simulink model "Open_Loop_shift"  (R2015a)
settings: Solver=ode3  StartTime=0.0  StopTime=300  FixedStep=0.01  MaxStep=0.01  RelTol=1e-3
values from neighbouring files (symbols this model uses):
  H0 = Periodic_Solution(1,4)    [Optimal_Entrainment_shiftworker.m]
  Ishift = 1000    [Optimal_Entrainment_shiftworker.m]
  n0 = Periodic_Solution(1,7)    [Optimal_Entrainment_shiftworker.m]
  Periodic_Solution = Periodic_Solution(1401:end,:)    [Optimal_Entrainment_shiftworker.m]
  shift = 12    [Optimal_Entrainment_shiftworker.m]
  tol = 0.01    [Optimal_Entrainment_shiftworker.m]
  x0 = Periodic_Solution(1,2)    [Optimal_Entrainment_shiftworker.m]
  xc0 = Periodic_Solution(1,3)    [Optimal_Entrainment_shiftworker.m]
settings Model: Creator=wangf7  LastModifiedBy=Jiawei Yin
settings OptimizationCC: ExpressionDepthLimit=2147483647
settings DebuggingCC: AlgebraicLoopMsg=none  ArtificialAlgebraicLoopMsg=none  UnderspecifiedInitializationDetection=Classic  MergeDetectMultiDrivingBlocksExec=none  SolverPrmCheckMsg=warning  StateNameClashWarn=warning

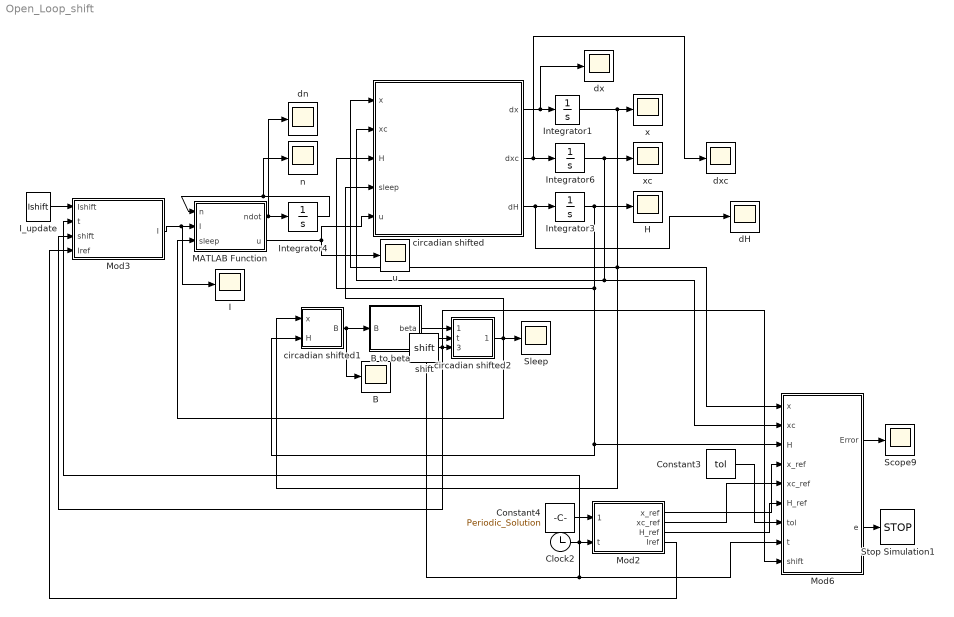
== system Open_Loop_shift ==
  B : Scope
      settings: TimeRange=auto  MaxDataPoints=5000  SaveName=B  YMin=-10  YMax=10  SampleTime=-1  DataFormat=Array
  "B to beta " : Subsystem
  Clock2 : Clock
  Constant3 : Constant  Value=tol
  Constant4 : Constant  Value=Periodic_Solution
  H : Scope
      settings: TimeRange=auto  MaxDataPoints=5000  SaveName=H  YMin=0.08394  YMax=0.57854  SampleTime=-1  DataFormat=Array
  I : Scope
      settings: TimeRange=auto  MaxDataPoints=5000  SaveName=I  YMin=-125.00000  YMax=1125.00000  SampleTime=-1  DataFormat=Array
  I_update : Constant  Value=Ishift
  Integrator1 : Integrator  InitialCondition=x0
  Integrator3 : Integrator  InitialCondition=H0
  Integrator4 : Integrator  InitialCondition=n0
  Integrator6 : Integrator  InitialCondition=xc0
  MATLAB Function : MATLAB Function  TreatAsAtomicUnit=on
      settings: PermitHierarchicalResolution=ParametersOnly
  Mod2 : MATLAB Function  TreatAsAtomicUnit=on
      settings: PermitHierarchicalResolution=ParametersOnly
  Mod3 : MATLAB Function  TreatAsAtomicUnit=on
      settings: PermitHierarchicalResolution=ParametersOnly
  Mod6 : MATLAB Function  TreatAsAtomicUnit=on
      settings: PermitHierarchicalResolution=ParametersOnly
  Scope9 : Scope
      settings: TimeRange=auto  MaxDataPoints=5000  SaveName=Error  YMin=0.00087  YMax=0.09507  SampleTime=-1  DataFormat=Array
  Sleep : Scope
      settings: TimeRange=auto  MaxDataPoints=5000  SaveName=Sleep  YMin=-0.125  YMax=1.125  SampleTime=-1  DataFormat=Array
  Stop Simulation1 : Stop
  circadian shifted : MATLAB Function  TreatAsAtomicUnit=on
      settings: PermitHierarchicalResolution=ParametersOnly
  circadian shifted1 : MATLAB Function  TreatAsAtomicUnit=on
      settings: PermitHierarchicalResolution=ParametersOnly
  circadian shifted2 : MATLAB Function  TreatAsAtomicUnit=on
      settings: PermitHierarchicalResolution=ParametersOnly
  dH : Scope
      settings: TimeRange=auto  MaxDataPoints=5000  SaveName=dH  YMin=0.03966  YMax=0.05966  SampleTime=-1  DataFormat=Array
  dn : Scope
      settings: TimeRange=auto  MaxDataPoints=5000  SaveName=dn  YMin=-10  YMax=10  SampleTime=-1  DataFormat=Array
  dx : Scope
      settings: TimeRange=auto  MaxDataPoints=5000  SaveName=dx  YMin=-10  YMax=10  SampleTime=-1  DataFormat=Array
  dxc : Scope
      settings: TimeRange=auto  MaxDataPoints=5000  SaveName=dxc  YMin=-10  YMax=10  SampleTime=-1  DataFormat=Array
  n : Scope
      settings: TimeRange=auto  MaxDataPoints=5000  SaveName=n  YMin=-10  YMax=10  SampleTime=-1  DataFormat=Array
  shift : Constant  Value=shift
  u : Scope
      settings: TimeRange=auto  MaxDataPoints=5000  SaveName=u  YMin=-0.12852  YMax=1.15668  SampleTime=-1  DataFormat=Array
  x : Scope
      settings: TimeRange=auto  MaxDataPoints=5000  SaveName=x  YMin=-0.56951  YMax=1.25946  SampleTime=-1  DataFormat=Array
  xc : Scope
      settings: TimeRange=auto  MaxDataPoints=5000  SaveName=xc  YMin=-1.29593  YMax=1.31086  SampleTime=-1  DataFormat=Array
  wires:
  circadian shifted/1(dx) -> Integrator1/1, dx/1
  Integrator1/1 -> circadian shifted1/1(x), Mod6/1(x), circadian shifted/1(x), x/1
  Integrator6/1 -> Mod6/2(xc), circadian shifted/2(xc), xc/1
  Constant4/1 -> Mod2/1(Periodic_Solution)
  Clock2/1 -> Mod6/8(t), circadian shifted2/2(t), Mod2/2(t), Mod3/2(t)
  Mod6/2(e) -> Stop Simulation1/1
  Mod6/1(Error) -> Scope9/1
  Mod2/3(H_ref) -> Mod6/6(H_ref)
  Constant3/1 -> Mod6/7(tol)
  circadian shifted/2(dxc) -> dxc/1, Integrator6/1
  Integrator3/1 -> circadian shifted1/2(H), Mod6/3(H), circadian shifted/3(H), H/1
  Mod2/1(x_ref) -> Mod6/4(x_ref)
  Mod2/2(xc_ref) -> Mod6/5(xc_ref)
  I_update/1 -> Mod3/1(Ishift)
  circadian shifted/3(dH) -> dH/1, Integrator3/1
  Mod3/1(I) -> I/1, MATLAB Function/2(I)
  MATLAB Function/2(u) -> circadian shifted/5(u), u/1
  MATLAB Function/1(ndot) -> dn/1, Integrator4/1
  Integrator4/1 -> n/1, MATLAB Function/1(n)
  circadian shifted1/1(B) -> B/1, "B to beta "/1(B)
  "B to beta "/1(beta) -> circadian shifted2/1(Sleep)
  Mod2/4(Iref) -> Mod3/4(Iref)
  circadian shifted2/1(sleep) -> Sleep/1, MATLAB Function/3(sleep), circadian shifted/4(sleep)
  shift/1 -> Mod3/3(shift), Mod6/9(shift), circadian shifted2/3(shift_time)

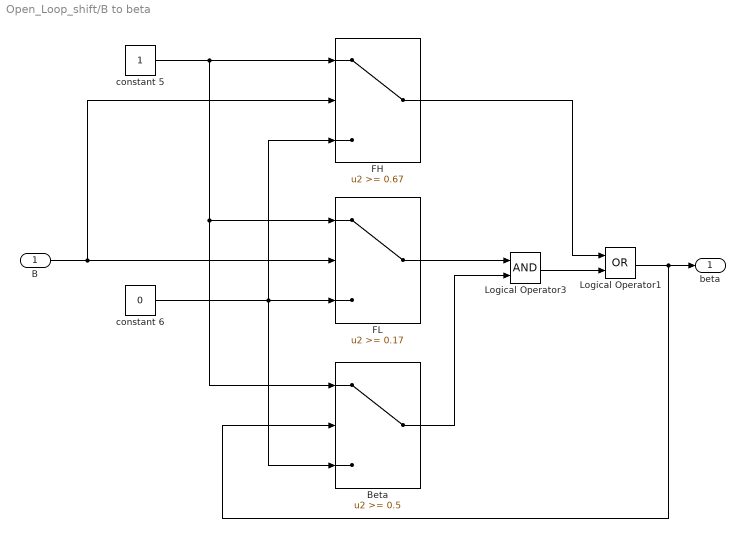
== system Open_Loop_shift/B to beta  ==
  B : Inport
  Beta : Switch  Threshold=0.5
  FH : Switch  Threshold=0.67
  FL : Switch  Threshold=0.17
  Logical Operator1 : Logic  Operator=OR  AllPortsSameDT=off  OutDataTypeStr=boolean
  Logical Operator3 : Logic  AllPortsSameDT=off  OutDataTypeStr=boolean
  constant 5 : Constant
  constant 6 : Constant  Value=0
  beta : Outport
  wires:
  constant 5/1 -> Beta/1, FL/1, FH/1
  constant 6/1 -> Beta/3, FH/3, FL/3
  B/1 -> FH/2, FL/2
  Logical Operator1/1 -> Beta/2, beta/1
  FL/1 -> Logical Operator3/1
  Beta/1 -> Logical Operator3/2
  Logical Operator3/1 -> Logical Operator1/2
  FH/1 -> Logical Operator1/1

== matlab function Open_Loop_shift/circadian shifted1 ==
  data: x input; H input; B output
function B = fcn(x,H)
%#eml
B=H-0.1333*x;

== matlab function Open_Loop_shift/circadian shifted2 ==
  data: Sleep input; t input; sleep output; shift_time input
function sleep = fcn(Sleep,t,shift_time)
%#eml
if t<shift_time
    sleep=0;
elseif Sleep
    sleep=1;
else
    sleep=0;
end

== matlab function Open_Loop_shift/MATLAB Function ==
  data: n input; I input; ndot output; u output; sleep input
function [ndot,u] = fcn(n,I,sleep)
G=33.75;
alpha0=0.05;
beta=0.0075;
I0=9500;

alpha=alpha0*(I/I0)^0.5;
u=G*alpha*(1-n)*(1-sleep);
ndot=60*[alpha*(1-n)*(1-sleep)-beta*n];

== matlab function Open_Loop_shift/circadian shifted ==
  data: x input; xc input; H input; sleep input; u input; dx output; dxc output; dH output
function [dx,dxc,dH] = fcn(x,xc,H,sleep,u)
%#eml

tr=18.2;
td=4.2;

q = 1/3;
taux = 24.2;
k = 0.55;
mu=0.13;

B = u*(1-0.4*x)*(1-0.4*xc)*(1-sleep);

dx = (pi/12)*(xc + B  + mu*(1/3*x + 4/3*x^3 - 256/105*x^7));
dxc = (pi/12)*(q*B *xc - (24/(taux*0.99729))^2*x - k*B*x);
dH = (1-sleep)*(1-H)/tr-(H*sleep)/td;

== matlab function Open_Loop_shift/Mod2 ==
  data: Periodic_Solution input; x_ref output; xc_ref output; t input; H_ref output; Iref output
function [x_ref,xc_ref,H_ref,Iref] = fcn(Periodic_Solution,t)
%#codegen
x_ref=interp1q(Periodic_Solution(:,1),Periodic_Solution(:,2),t);
xc_ref=interp1q(Periodic_Solution(:,1),Periodic_Solution(:,3),t);
H_ref=interp1q(Periodic_Solution(:,1),Periodic_Solution(:,4),t);
Iref=interp1q(Periodic_Solution(:,1),Periodic_Solution(:,5),t);

== matlab function Open_Loop_shift/Mod6 ==
  data: Error output; x input; xc input; H input; x_ref input; xc_ref input; e output; H_ref input; tol input; t input; shift input
function [Error,e] = fcn(x,xc,H,x_ref,xc_ref,H_ref,tol,t,shift)
%#codegen
Error=(H-H_ref)^2+(x-x_ref)^2+(xc-xc_ref)^2;
e=Error<tol && t>=shift;

== matlab function Open_Loop_shift/Mod3 ==
  data: Ishift input; I output; t input; shift input; Iref input
function I  = fcn(Ishift,t,shift,Iref)
%#codegen
if t<shift
    I=Ishift;
else
    I=Iref;
end
